simulink model "Fu02"  (Simulink 5.0)
settings: Solver=ode23tb  StartTime=0.0  StopTime=inf  MaxStep=1/90000  MinStep=1/100000000  RelTol=1e-6
undefined symbols (not defined in the file or in its folder): get, RFS01
libraries: simulink x2, commcontsrc2 x2, dspsnks4 x1
settings Model: LastModifiedBy=efst

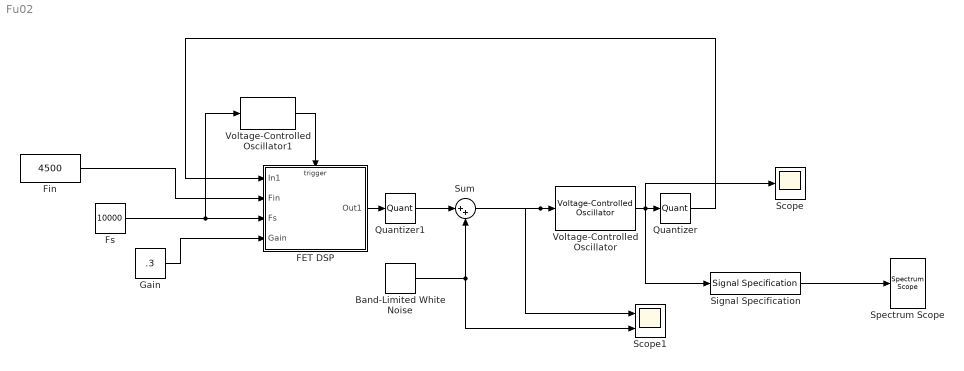
== system Fu02 ==
  Band-Limited White Noise : simulink/Sources/Band-Limited White Noise  Cov=[0.00]  Ts=2/10000  seed=[23341]
  FET DSP : Subsystem  TreatAsAtomicUnit=on
  Fin : Constant  Value=4500
  Fs : Constant  Value=10000
  Gain : Constant  Value=.3
  Quantizer : Quantizer  QuantizationInterval=2/(2^8)
  Quantizer1 : Quantizer  QuantizationInterval=0.001
  Scope : Scope
      settings: TimeRange=0.0009417969485778867  YMin=-1  YMax=1
  Scope1 : Scope  NumInputPorts=2
      settings: TimeRange=0.02  YMin=0~-1  YMax=1100~1
  Signal Specification : simulink/Signal Attributes/Signal Specification  D=1  Ts=1/10000  DataType=auto  OutDataType=sfix(16)  OutScaling=2^0
      settings: SignalType=auto  SamplingMode=sample-based
  Spectrum Scope : dspsnks4/Spectrum Scope  ScopeProperties=on  Domain=Frequency  HorizSpan=1  UseBuffer=on  BufferSize=1024  Overlap=64  inpFftLenInherit=on  FFTlength=1024  numAvg=12  DisplayProperties=off  AxisGrid=on  Memory=off  FrameNumber=on  AxisLegend=off  AxisZoom=off  OpenScopeAtSimStart=on  OpenScopeImmediately=off  FigPos=get(0,'defaultfigureposition')  AxisProperties=off  XUnits=Hertz  XRange=[0...Fs/2]  InheritXIncr=on  XIncr=1.0  XLabel=Samples  YUnits=dB  YLabel=Magnitude, dB  LineProperties=off
      settings: YMin=-99.5072296404508  YMax=27.4621508189047
  Sum : Sum  Inputs=|++  SaturateOnIntegerOverflow=on
  Voltage-Controlled Oscillator : commcontsrc2/Voltage-Controlled Oscillator  Ac=1  Fc=0  Kc=1  Ph=0
  Voltage-Controlled Oscillator1 : commcontsrc2/Voltage-Controlled Oscillator  Ac=1  Fc=0  Kc=1  Ph=0
  wires:
  Voltage-Controlled Oscillator/1 -> Signal Specification/1, Quantizer/1, Scope/1
  Fin/1 -> FET DSP/2(Fin)
  Fs/1 -> FET DSP/3(Fs), Voltage-Controlled Oscillator1/1
  Gain/1 -> FET DSP/4(Gain)
  Voltage-Controlled Oscillator1/1 -> FET DSP/Trigger
  Quantizer/1 -> FET DSP/1(In1)
  FET DSP/1(Out1) -> Quantizer1/1
  Quantizer1/1 -> Sum/1
  Sum/1 -> Voltage-Controlled Oscillator/1, Scope1/1
  Band-Limited White Noise/1 -> Sum/2, Scope1/2
  Signal Specification/1 -> Spectrum Scope/1

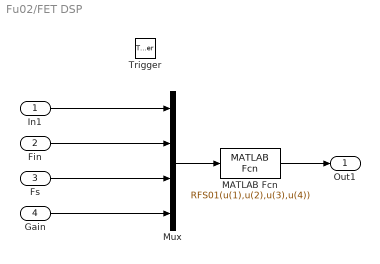
== system Fu02/FET DSP ==
  In1 : Inport
  Fin : Inport  Port=2
  Fs : Inport  Port=3
  Gain : Inport  Port=4
  Trigger : TriggerPort
  MATLAB Fcn : MATLABFcn  MATLABFcn=RFS01(u(1),u(2),u(3),u(4))  OutputDimensions=1
  Mux : Mux
  Out1 : Outport
  wires:
  Fin/1 -> Mux/2
  Mux/1 -> MATLAB Fcn/1
  In1/1 -> Mux/1
  MATLAB Fcn/1 -> Out1/1
  Fs/1 -> Mux/3
  Gain/1 -> Mux/4
